simulink model "Linear_NonLinear_Model"  (R2023b)
settings: Solver=VariableStepAuto  StartTime=0.0  StopTime=400  RelTol=1e-3
undefined symbols (not defined in the file or in its folder): magnitude, P
libraries: vrlib x21
settings Model: Creator=pinki  LastModifiedBy=pinki

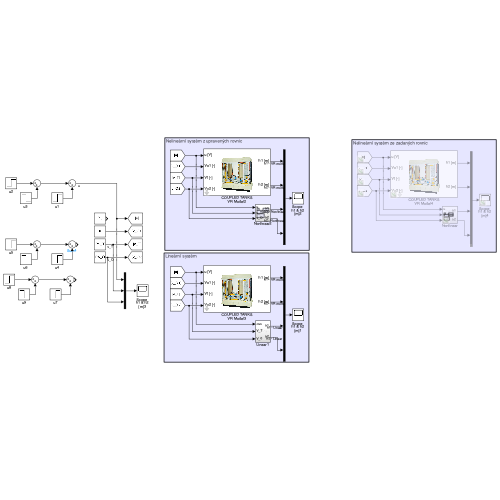
[thumbnail: Simulink's stored preview of the top-level diagram]
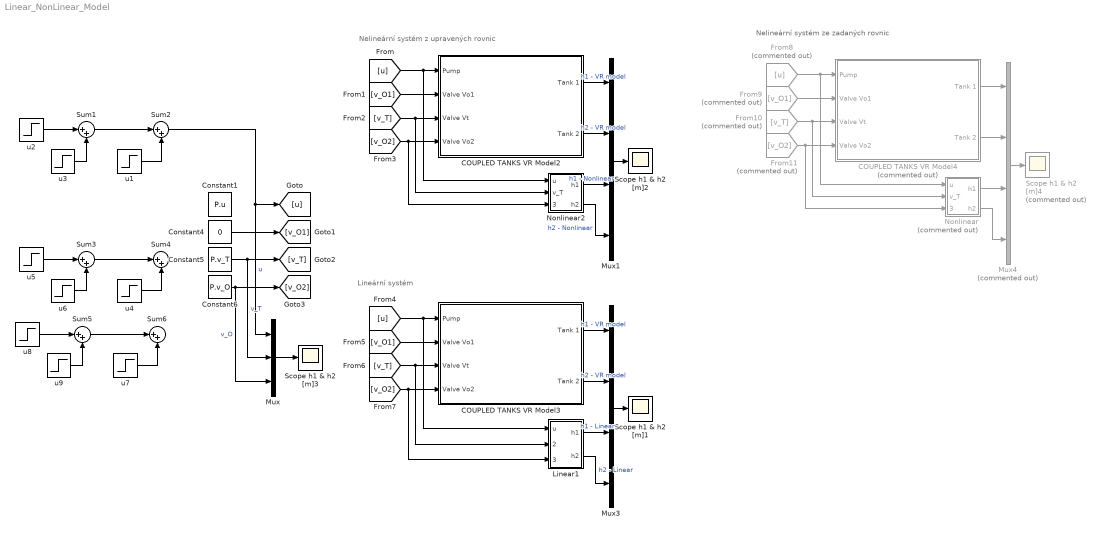
== system Linear_NonLinear_Model ==
  note: Lineární systém
  note: Nelineární systém z upravených rovnic
  note: Nelineární systém ze zadaných rovnic
  COUPLED TANKS VR Model2 : Subsystem  mask(Coupled Tanks (CT) in laboratory K26){showVR=off, sfcnParam1=P.h1, sfcnParam2=P.h2}
      mask prompts: showVR "Show VirtualWorld?"; sfcnParam1 "Initial fluid level in the left tank 1   h1(0)  [cm]"; sfcnParam2 "Initial fluid  level in the right tank 2   h2 (0) [cm]"
      mask help:
      | Coupled Tanks (CT) in laboratory K26 - Virtual Reality
      | Real-Time Workshop generated S-function.
      mask Help:
      | Couple Tanks in laboratory K26 - Virtual Reality. <br><br>
      | 
      | 
      | This is a&nbsp;virtual model of the Coupled Tanks apparatus in Laboratory of automatic control
      | theory&nbsp;26 (<a href="http://support.dce.felk.cvut.cz/lab26/" target="_blank">http://support.dce.felk.cvut.cz/lab26/</a>),
      | which consists of a&nbsp;gear-pump, two tanks (left and right), inflow and outflow pipes and transfer (V<sub>t</sub>) and
      | output valves (V<sub>o1</sub>, V<sub>o2</sub>). The&nbsp;left tank is filled with the&nbsp;fluid by the&nbsp;gear-pump
      | controller by the&nbsp;voltage&nbsp;<em>u</em>&nbsp;[V]. The&nbsp;fluid can drain from the&nbsp;left tank through
      | the&nbsp;valve&nbsp;<em>v</em><sub>o1</sub>&nbsp;[%] or can drain to the&nbsp;right tank through the&nbsp;transfer
      | valve&nbsp;<em>v</em><sub>t</sub>&nbsp;[%]. The&nbsp;fluid drains away from the&nbsp;right tank through
      | the&nbsp;valve&nbsp;<em>v</em><sub>o2</sub>&nbsp;[%].<br><br>
      | 
      | The&nbsp;system input are the&nbsp;voltage of the&nbsp;motor of the&nbsp;gear-pump&nbsp;<em>u</em>&nbsp;[V]
      | and the&nbsp;opening of
      | the&nbsp;valves&nbsp;<em>v</em><sub>o1</sub>,&nbsp;<em>v</em><sub>t</sub>,&nbsp;<em>v</em><sub>o2</sub>&nbsp;[%].
      | The&nbsp;system outputs are the&nbsp;levels of the&nbsp;fluid in
      | the&nbsp;tanks&nbsp;<em>h</em><sub>1</sub>,&nbsp;<em>h</em><sub>2</sub>&nbsp;[cm].
      | The&nbsp;dynamics of the&nbsp;gear-pump is neglected. More information can be found on the&nbsp;website
      | <a href="http://support.dce.felk.cvut.cz/lab26/" target="_blank">http://support.dce.felk.cvut.cz/lab26/</a>.<br><br>
      | 
      | 
      | In the mask of the model, it can be set:
      | <ul>
      | <li>Initial fluid level in the left tank</li>
      | <li>Initial fluid level in the right tank.</li>
      | </ul><br><br>
      | 
      | 
      | Copyright: 2008, Jan Kricka, Jirka Roubal, Petr Husek.
      mask Callback showVR:
      | if strcmp('off',get_param(gcb,'showVR'))
      |     vrclose all;
      | else
      |     if exist('figureVR')==0
      |         figureVR = vrfigure;
      |     end
      |     if exist('worldVR')==0
      |         worldVR = vrworld('CoupledTanks_VR.WRL');
      |     end
      | 	if isvalid(figureVR)==0
      |         open(worldVR);
      |         figureVR = vrfigure(worldVR,[650 80 550 350]);
      | 	end
      | end
      mask Display:
      | image(imread('CoupledTanks_Image.jpg'));
      | port_label ('input',1,'u [V]');
      | port_label ('input',2,'Vo1 [-]');
      | port_label ('input',3,'Vt [-]');
      | port_label ('input',4,'Vo2 [-]');
      | port_label ('output',1,'h1 [m]');
      | port_label ('output',2,'h2 [m]');
  COUPLED TANKS VR Model3 : Subsystem  mask(Coupled Tanks (CT) in laboratory K26){showVR=off, sfcnParam1=P.h1, sfcnParam2=P.h2}
      mask prompts: showVR "Show VirtualWorld?"; sfcnParam1 "Initial fluid level in the left tank 1   h1(0)  [cm]"; sfcnParam2 "Initial fluid  level in the right tank 2   h2 (0) [cm]"
      mask help:
      | Coupled Tanks (CT) in laboratory K26 - Virtual Reality
      | Real-Time Workshop generated S-function.
      mask Help:
      | Couple Tanks in laboratory K26 - Virtual Reality. <br><br>
      | 
      | 
      | This is a&nbsp;virtual model of the Coupled Tanks apparatus in Laboratory of automatic control
      | theory&nbsp;26 (<a href="http://support.dce.felk.cvut.cz/lab26/" target="_blank">http://support.dce.felk.cvut.cz/lab26/</a>),
      | which consists of a&nbsp;gear-pump, two tanks (left and right), inflow and outflow pipes and transfer (V<sub>t</sub>) and
      | output valves (V<sub>o1</sub>, V<sub>o2</sub>). The&nbsp;left tank is filled with the&nbsp;fluid by the&nbsp;gear-pump
      | controller by the&nbsp;voltage&nbsp;<em>u</em>&nbsp;[V]. The&nbsp;fluid can drain from the&nbsp;left tank through
      | the&nbsp;valve&nbsp;<em>v</em><sub>o1</sub>&nbsp;[%] or can drain to the&nbsp;right tank through the&nbsp;transfer
      | valve&nbsp;<em>v</em><sub>t</sub>&nbsp;[%]. The&nbsp;fluid drains away from the&nbsp;right tank through
      | the&nbsp;valve&nbsp;<em>v</em><sub>o2</sub>&nbsp;[%].<br><br>
      | 
      | The&nbsp;system input are the&nbsp;voltage of the&nbsp;motor of the&nbsp;gear-pump&nbsp;<em>u</em>&nbsp;[V]
      | and the&nbsp;opening of
      | the&nbsp;valves&nbsp;<em>v</em><sub>o1</sub>,&nbsp;<em>v</em><sub>t</sub>,&nbsp;<em>v</em><sub>o2</sub>&nbsp;[%].
      | The&nbsp;system outputs are the&nbsp;levels of the&nbsp;fluid in
      | the&nbsp;tanks&nbsp;<em>h</em><sub>1</sub>,&nbsp;<em>h</em><sub>2</sub>&nbsp;[cm].
      | The&nbsp;dynamics of the&nbsp;gear-pump is neglected. More information can be found on the&nbsp;website
      | <a href="http://support.dce.felk.cvut.cz/lab26/" target="_blank">http://support.dce.felk.cvut.cz/lab26/</a>.<br><br>
      | 
      | 
      | In the mask of the model, it can be set:
      | <ul>
      | <li>Initial fluid level in the left tank</li>
      | <li>Initial fluid level in the right tank.</li>
      | </ul><br><br>
      | 
      | 
      | Copyright: 2008, Jan Kricka, Jirka Roubal, Petr Husek.
      mask Callback showVR:
      | if strcmp('off',get_param(gcb,'showVR'))
      |     vrclose all;
      | else
      |     if exist('figureVR')==0
      |         figureVR = vrfigure;
      |     end
      |     if exist('worldVR')==0
      |         worldVR = vrworld('CoupledTanks_VR.WRL');
      |     end
      | 	if isvalid(figureVR)==0
      |         open(worldVR);
      |         figureVR = vrfigure(worldVR,[650 80 550 350]);
      | 	end
      | end
      mask Display:
      | image(imread('CoupledTanks_Image.jpg'));
      | port_label ('input',1,'u [V]');
      | port_label ('input',2,'Vo1 [-]');
      | port_label ('input',3,'Vt [-]');
      | port_label ('input',4,'Vo2 [-]');
      | port_label ('output',1,'h1 [m]');
      | port_label ('output',2,'h2 [m]');
  COUPLED TANKS VR Model4 : Subsystem  Commented=on  mask(Coupled Tanks (CT) in laboratory K26){showVR=off, sfcnParam1=P.h1, sfcnParam2=P.h2}
      mask prompts: showVR "Show VirtualWorld?"; sfcnParam1 "Initial fluid level in the left tank 1   h1(0)  [cm]"; sfcnParam2 "Initial fluid  level in the right tank 2   h2 (0) [cm]"
      mask help:
      | Coupled Tanks (CT) in laboratory K26 - Virtual Reality
      | Real-Time Workshop generated S-function.
      mask Help:
      | Couple Tanks in laboratory K26 - Virtual Reality. <br><br>
      | 
      | 
      | This is a&nbsp;virtual model of the Coupled Tanks apparatus in Laboratory of automatic control
      | theory&nbsp;26 (<a href="http://support.dce.felk.cvut.cz/lab26/" target="_blank">http://support.dce.felk.cvut.cz/lab26/</a>),
      | which consists of a&nbsp;gear-pump, two tanks (left and right), inflow and outflow pipes and transfer (V<sub>t</sub>) and
      | output valves (V<sub>o1</sub>, V<sub>o2</sub>). The&nbsp;left tank is filled with the&nbsp;fluid by the&nbsp;gear-pump
      | controller by the&nbsp;voltage&nbsp;<em>u</em>&nbsp;[V]. The&nbsp;fluid can drain from the&nbsp;left tank through
      | the&nbsp;valve&nbsp;<em>v</em><sub>o1</sub>&nbsp;[%] or can drain to the&nbsp;right tank through the&nbsp;transfer
      | valve&nbsp;<em>v</em><sub>t</sub>&nbsp;[%]. The&nbsp;fluid drains away from the&nbsp;right tank through
      | the&nbsp;valve&nbsp;<em>v</em><sub>o2</sub>&nbsp;[%].<br><br>
      | 
      | The&nbsp;system input are the&nbsp;voltage of the&nbsp;motor of the&nbsp;gear-pump&nbsp;<em>u</em>&nbsp;[V]
      | and the&nbsp;opening of
      | the&nbsp;valves&nbsp;<em>v</em><sub>o1</sub>,&nbsp;<em>v</em><sub>t</sub>,&nbsp;<em>v</em><sub>o2</sub>&nbsp;[%].
      | The&nbsp;system outputs are the&nbsp;levels of the&nbsp;fluid in
      | the&nbsp;tanks&nbsp;<em>h</em><sub>1</sub>,&nbsp;<em>h</em><sub>2</sub>&nbsp;[cm].
      | The&nbsp;dynamics of the&nbsp;gear-pump is neglected. More information can be found on the&nbsp;website
      | <a href="http://support.dce.felk.cvut.cz/lab26/" target="_blank">http://support.dce.felk.cvut.cz/lab26/</a>.<br><br>
      | 
      | 
      | In the mask of the model, it can be set:
      | <ul>
      | <li>Initial fluid level in the left tank</li>
      | <li>Initial fluid level in the right tank.</li>
      | </ul><br><br>
      | 
      | 
      | Copyright: 2008, Jan Kricka, Jirka Roubal, Petr Husek.
      mask Callback showVR:
      | if strcmp('off',get_param(gcb,'showVR'))
      |     vrclose all;
      | else
      |     if exist('figureVR')==0
      |         figureVR = vrfigure;
      |     end
      |     if exist('worldVR')==0
      |         worldVR = vrworld('CoupledTanks_VR.WRL');
      |     end
      | 	if isvalid(figureVR)==0
      |         open(worldVR);
      |         figureVR = vrfigure(worldVR,[650 80 550 350]);
      | 	end
      | end
      mask Display:
      | image(imread('CoupledTanks_Image.jpg'));
      | port_label ('input',1,'u [V]');
      | port_label ('input',2,'Vo1 [-]');
      | port_label ('input',3,'Vt [-]');
      | port_label ('input',4,'Vo2 [-]');
      | port_label ('output',1,'h1 [m]');
      | port_label ('output',2,'h2 [m]');
  Constant1 : Constant  Value=P.u
  Constant4 : Constant  Value=0
  Constant5 : Constant  Value=P.v_T
  Constant6 : Constant  Value=P.v_O
  From10 : From  Commented=on  GotoTag=v_T
  From11 : From  Commented=on  GotoTag=v_O2
  From8 : From  Commented=on  GotoTag=u
  From9 : From  Commented=on  GotoTag=v_O1
  Linear1 : Subsystem
  Mux : Mux  Inputs=3
  Mux1 : Mux
  Mux3 : Mux
  Mux4 : Mux  Commented=on
  Nonlinear : Subsystem  Commented=on
  Nonlinear2 : Subsystem
  Scope h1 & h2 [m]1 : Scope
  Scope h1 & h2 [m]2 : Scope
  Scope h1 & h2 [m]3 : Scope
  Scope h1 & h2 [m]4 : Scope  Commented=on
  Sum{1..6} (6 alike) : Sum  Inputs=|++
  u1 : Step  Time=300  After=2  SampleTime=0
  u2 : Step  Time=100  Before=P.u  After=P.u+0.5  SampleTime=0
  u3 : Step  Time=200  After=-1  SampleTime=0
  u4 : Step  Time=300  After=0.4  SampleTime=0
  u5 : Step  Time=100  Before=P.v_T  After=P.v_T+0.1  SampleTime=0
  u6 : Step  Time=200  After=-0.2  SampleTime=0
  u7 : Step  Time=300  After=0.4  SampleTime=0
  u8 : Step  Time=100  Before=P.v_O  After=P.v_O+0.1  SampleTime=0
  u9 : Step  Time=200  After=-0.2  SampleTime=0
  wires:
  [v_O2] -> Nonlinear2/3(v_O), COUPLED TANKS VR Model2/4(Valve Vo2)
  COUPLED TANKS VR Model2/1(Tank 1) -> Mux1/1  "h1 - VR model"
  Sum1/1 -> Sum2/1
  u1/1 -> Sum2/2
  [v_O1] -> COUPLED TANKS VR Model2/2(Valve Vo1)
  u3/1 -> Sum1/2
  [v_T] -> COUPLED TANKS VR Model2/3(Valve Vt), Nonlinear2/2(v_T)
  Mux1/1 -> Scope h1 & h2 [m]2/1
  COUPLED TANKS VR Model2/2(Tank 2) -> Mux1/2  "h2 - VR model"
  u2/1 -> Sum1/1
  Nonlinear2/1(h1) -> Mux1/3  "h1 - Nonlinear"
  Nonlinear2/2(h2) -> Mux1/4  "h2 - Nonlinear"
  [u] -> Nonlinear2/1(u), COUPLED TANKS VR Model2/1(Pump)
  Constant4/1 -> [v_O1]
  [v_T] -> Linear1/2(V_T), COUPLED TANKS VR Model3/3(Valve Vt)
  COUPLED TANKS VR Model3/1(Tank 1) -> Mux3/1  "h1 - VR model"
  Linear1/2(h2) -> Mux3/4  "h2 - Linear"
  Linear1/1(h1) -> Mux3/3  "h1 - Linear"
  Mux3/1 -> Scope h1 & h2 [m]1/1
  COUPLED TANKS VR Model3/2(Tank 2) -> Mux3/2  "h2 - VR model"
  [u] -> Linear1/1(u), COUPLED TANKS VR Model3/1(Pump)
  [v_O2] -> Linear1/3(V_0), COUPLED TANKS VR Model3/4(Valve Vo2)
  [v_O1] -> COUPLED TANKS VR Model3/2(Valve Vo1)
  Mux4/1 -> Scope h1 & h2 [m]4/1
  COUPLED TANKS VR Model4/2(Tank 2) -> Mux4/2
  Nonlinear/1(h1) -> Mux4/3
  Nonlinear/2(h2) -> Mux4/4
  From8/1 -> Nonlinear/1(u), COUPLED TANKS VR Model4/1(Pump)
  COUPLED TANKS VR Model4/1(Tank 1) -> Mux4/1
  From11/1 -> Nonlinear/3(v_O), COUPLED TANKS VR Model4/4(Valve Vo2)
  From10/1 -> Nonlinear/2(v_T), COUPLED TANKS VR Model4/3(Valve Vt)
  From9/1 -> COUPLED TANKS VR Model4/2(Valve Vo1)
  Sum3/1 -> Sum4/1
  u4/1 -> Sum4/2
  u6/1 -> Sum3/2
  u5/1 -> Sum3/1
  Mux/1 -> Scope h1 & h2 [m]3/1
  Sum5/1 -> Sum6/1
  u7/1 -> Sum6/2
  u8/1 -> Sum5/1
  u9/1 -> Sum5/2
  Constant6/1 -> Mux/3, [v_O2]  "v_O"
  Constant5/1 -> Mux/2, [v_T]  "v_T"
  Sum2/1 -> [u], Mux/1  "u"

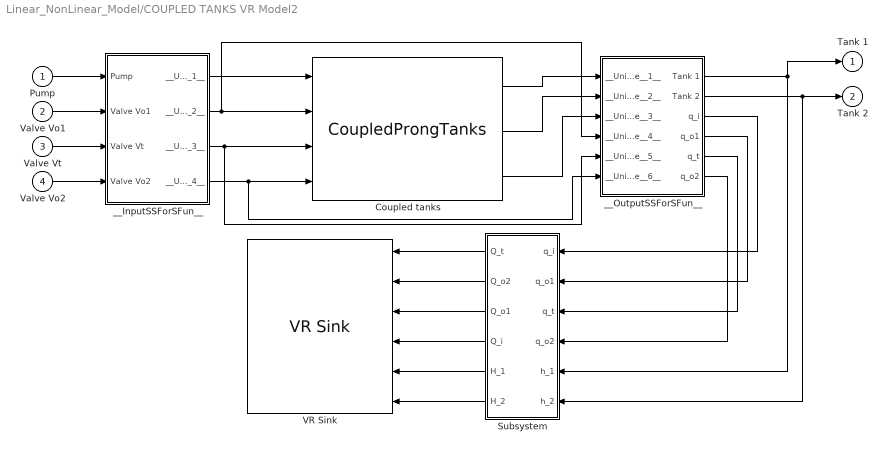
== system Linear_NonLinear_Model/COUPLED TANKS VR Model2 ==
  Pump : Inport
  Valve Vo1 : Inport  Port=2
  Valve Vt : Inport  Port=3
  Valve Vo2 : Inport  Port=4
  Coupled tanks : M-S-Function  FunctionName=CoupledProngTanks  Parameters=h10 h20  mask{h10=sfcnParam1, h20=sfcnParam2}
      mask prompts: h10 "h1_init"; h20 "h2_init"
      mask Display:
      | port_label('input',1,'Pump');
      | port_label('input',2,'Valve Vo1');
      | port_label('input',3,'Valve Vt');
      | port_label('input',4,'Valve Vo2');
      | port_label('output',1,'Tank 1');
      | port_label('output',2,'Tank 2');
      | port_label('output',3,'q_i');
  Subsystem : Subsystem
  VR Sink : vrlib/VR Sink  InstantiateOnLoad=on  SampleTime=-1  ViewEnable=on  RemoteChange=off  RemoteView=on  FieldsWritten=Valve_t.rotation.4.1.double#Valve_o2.rotation.4.1.double#Valve_o1.rotation.4.1.double#Pump.rotation.4.1.double#water1.scale.3.1.double#water2.scale.3.1.double  WorldFileName=CoupledTanks_VR.WRL  AutoView=off  VideoDimensions=[]  AllowVariableSize=off
  __InputSSForSFun__ : Subsystem
  __OutputSSForSFun__ : Subsystem
  Tank 1 : Outport  OutDataTypeStr=double  PortDimensions=1  SampleTime=[-1 0]
  Tank 2 : Outport  Port=2  OutDataTypeStr=double  PortDimensions=1  SampleTime=[-1 0]
  wires:
  __OutputSSForSFun__/6(q_o2) -> Subsystem/4(q_o2)
  __OutputSSForSFun__/5(q_t) -> Subsystem/3(q_t)
  __OutputSSForSFun__/4(q_o1) -> Subsystem/2(q_o1)
  __OutputSSForSFun__/3(q_i) -> Subsystem/1(q_i)
  Subsystem/2(Q_o2) -> VR Sink/2
  Subsystem/3(Q_o1) -> VR Sink/3
  Subsystem/4(Q_i) -> VR Sink/4
  Subsystem/1(Q_t) -> VR Sink/1
  Subsystem/6(H_2) -> VR Sink/6
  Subsystem/5(H_1) -> VR Sink/5
  __OutputSSForSFun__/2(Tank 2) -> Subsystem/6(h_2), Tank 2/1
  __OutputSSForSFun__/1(Tank 1) -> Tank 1/1, Subsystem/5(h_1)
  __InputSSForSFun__/4(__UniqueOutportName__4__) -> __OutputSSForSFun__/6(__UniqueInportName__6__), Coupled tanks/4
  __InputSSForSFun__/3(__UniqueOutportName__3__) -> __OutputSSForSFun__/5(__UniqueInportName__5__), Coupled tanks/3
  Coupled tanks/2 -> __OutputSSForSFun__/2(__UniqueInportName__2__)
  Coupled tanks/1 -> __OutputSSForSFun__/1(__UniqueInportName__1__)
  __InputSSForSFun__/2(__UniqueOutportName__2__) -> __OutputSSForSFun__/4(__UniqueInportName__4__), Coupled tanks/2
  __InputSSForSFun__/1(__UniqueOutportName__1__) -> Coupled tanks/1
  Valve Vo2/1 -> __InputSSForSFun__/4(Valve Vo2)
  Valve Vt/1 -> __InputSSForSFun__/3(Valve Vt)
  Valve Vo1/1 -> __InputSSForSFun__/2(Valve Vo1)
  Pump/1 -> __InputSSForSFun__/1(Pump)
  Coupled tanks/3 -> __OutputSSForSFun__/3(__UniqueInportName__3__)

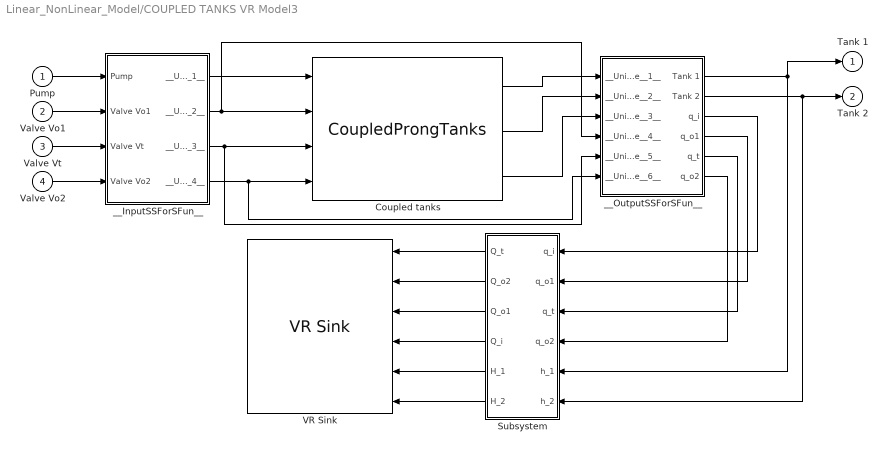
== system Linear_NonLinear_Model/COUPLED TANKS VR Model3 ==
  Pump : Inport
  Valve Vo1 : Inport  Port=2
  Valve Vt : Inport  Port=3
  Valve Vo2 : Inport  Port=4
  Coupled tanks : M-S-Function  FunctionName=CoupledProngTanks  Parameters=h10 h20  mask{h10=sfcnParam1, h20=sfcnParam2}
      mask prompts: h10 "h1_init"; h20 "h2_init"
      mask Display:
      | port_label('input',1,'Pump');
      | port_label('input',2,'Valve Vo1');
      | port_label('input',3,'Valve Vt');
      | port_label('input',4,'Valve Vo2');
      | port_label('output',1,'Tank 1');
      | port_label('output',2,'Tank 2');
      | port_label('output',3,'q_i');
  Subsystem : Subsystem
  VR Sink : vrlib/VR Sink  InstantiateOnLoad=on  SampleTime=-1  ViewEnable=on  RemoteChange=off  RemoteView=on  FieldsWritten=Valve_t.rotation.4.1.double#Valve_o2.rotation.4.1.double#Valve_o1.rotation.4.1.double#Pump.rotation.4.1.double#water1.scale.3.1.double#water2.scale.3.1.double  WorldFileName=CoupledTanks_VR.WRL  AutoView=off  VideoDimensions=[]  AllowVariableSize=off
  __InputSSForSFun__ : Subsystem
  __OutputSSForSFun__ : Subsystem
  Tank 1 : Outport  OutDataTypeStr=double  PortDimensions=1  SampleTime=[-1 0]
  Tank 2 : Outport  Port=2  OutDataTypeStr=double  PortDimensions=1  SampleTime=[-1 0]
  wires:
  __OutputSSForSFun__/6(q_o2) -> Subsystem/4(q_o2)
  __OutputSSForSFun__/5(q_t) -> Subsystem/3(q_t)
  __OutputSSForSFun__/4(q_o1) -> Subsystem/2(q_o1)
  __OutputSSForSFun__/3(q_i) -> Subsystem/1(q_i)
  Subsystem/2(Q_o2) -> VR Sink/2
  Subsystem/3(Q_o1) -> VR Sink/3
  Subsystem/4(Q_i) -> VR Sink/4
  Subsystem/1(Q_t) -> VR Sink/1
  Subsystem/6(H_2) -> VR Sink/6
  Subsystem/5(H_1) -> VR Sink/5
  __OutputSSForSFun__/2(Tank 2) -> Subsystem/6(h_2), Tank 2/1
  __OutputSSForSFun__/1(Tank 1) -> Tank 1/1, Subsystem/5(h_1)
  __InputSSForSFun__/4(__UniqueOutportName__4__) -> __OutputSSForSFun__/6(__UniqueInportName__6__), Coupled tanks/4
  __InputSSForSFun__/3(__UniqueOutportName__3__) -> __OutputSSForSFun__/5(__UniqueInportName__5__), Coupled tanks/3
  Coupled tanks/2 -> __OutputSSForSFun__/2(__UniqueInportName__2__)
  Coupled tanks/1 -> __OutputSSForSFun__/1(__UniqueInportName__1__)
  __InputSSForSFun__/2(__UniqueOutportName__2__) -> __OutputSSForSFun__/4(__UniqueInportName__4__), Coupled tanks/2
  __InputSSForSFun__/1(__UniqueOutportName__1__) -> Coupled tanks/1
  Valve Vo2/1 -> __InputSSForSFun__/4(Valve Vo2)
  Valve Vt/1 -> __InputSSForSFun__/3(Valve Vt)
  Valve Vo1/1 -> __InputSSForSFun__/2(Valve Vo1)
  Pump/1 -> __InputSSForSFun__/1(Pump)
  Coupled tanks/3 -> __OutputSSForSFun__/3(__UniqueInportName__3__)

== system Linear_NonLinear_Model/COUPLED TANKS VR Model4 ==
  Pump : Inport
  Valve Vo1 : Inport  Port=2
  Valve Vt : Inport  Port=3
  Valve Vo2 : Inport  Port=4
  Coupled tanks : M-S-Function  FunctionName=CoupledProngTanks  Parameters=h10 h20  mask{h10=sfcnParam1, h20=sfcnParam2}
      mask prompts: h10 "h1_init"; h20 "h2_init"
      mask Display:
      | port_label('input',1,'Pump');
      | port_label('input',2,'Valve Vo1');
      | port_label('input',3,'Valve Vt');
      | port_label('input',4,'Valve Vo2');
      | port_label('output',1,'Tank 1');
      | port_label('output',2,'Tank 2');
      | port_label('output',3,'q_i');
  Subsystem : Subsystem
  VR Sink : vrlib/VR Sink  InstantiateOnLoad=on  SampleTime=-1  ViewEnable=on  RemoteChange=off  RemoteView=on  FieldsWritten=Valve_t.rotation.4.1.double#Valve_o2.rotation.4.1.double#Valve_o1.rotation.4.1.double#Pump.rotation.4.1.double#water1.scale.3.1.double#water2.scale.3.1.double  WorldFileName=CoupledTanks_VR.WRL  AutoView=off  VideoDimensions=[]  AllowVariableSize=off
  __InputSSForSFun__ : Subsystem
  __OutputSSForSFun__ : Subsystem
  Tank 1 : Outport  OutDataTypeStr=double  PortDimensions=1  SampleTime=[-1 0]
  Tank 2 : Outport  Port=2  OutDataTypeStr=double  PortDimensions=1  SampleTime=[-1 0]
  wires:
  __OutputSSForSFun__/6(q_o2) -> Subsystem/4(q_o2)
  __OutputSSForSFun__/5(q_t) -> Subsystem/3(q_t)
  __OutputSSForSFun__/4(q_o1) -> Subsystem/2(q_o1)
  __OutputSSForSFun__/3(q_i) -> Subsystem/1(q_i)
  Subsystem/2(Q_o2) -> VR Sink/2
  Subsystem/3(Q_o1) -> VR Sink/3
  Subsystem/4(Q_i) -> VR Sink/4
  Subsystem/1(Q_t) -> VR Sink/1
  Subsystem/6(H_2) -> VR Sink/6
  Subsystem/5(H_1) -> VR Sink/5
  __OutputSSForSFun__/2(Tank 2) -> Subsystem/6(h_2), Tank 2/1
  __OutputSSForSFun__/1(Tank 1) -> Tank 1/1, Subsystem/5(h_1)
  __InputSSForSFun__/4(__UniqueOutportName__4__) -> __OutputSSForSFun__/6(__UniqueInportName__6__), Coupled tanks/4
  __InputSSForSFun__/3(__UniqueOutportName__3__) -> __OutputSSForSFun__/5(__UniqueInportName__5__), Coupled tanks/3
  Coupled tanks/2 -> __OutputSSForSFun__/2(__UniqueInportName__2__)
  Coupled tanks/1 -> __OutputSSForSFun__/1(__UniqueInportName__1__)
  __InputSSForSFun__/2(__UniqueOutportName__2__) -> __OutputSSForSFun__/4(__UniqueInportName__4__), Coupled tanks/2
  __InputSSForSFun__/1(__UniqueOutportName__1__) -> Coupled tanks/1
  Valve Vo2/1 -> __InputSSForSFun__/4(Valve Vo2)
  Valve Vt/1 -> __InputSSForSFun__/3(Valve Vt)
  Valve Vo1/1 -> __InputSSForSFun__/2(Valve Vo1)
  Pump/1 -> __InputSSForSFun__/1(Pump)
  Coupled tanks/3 -> __OutputSSForSFun__/3(__UniqueInportName__3__)

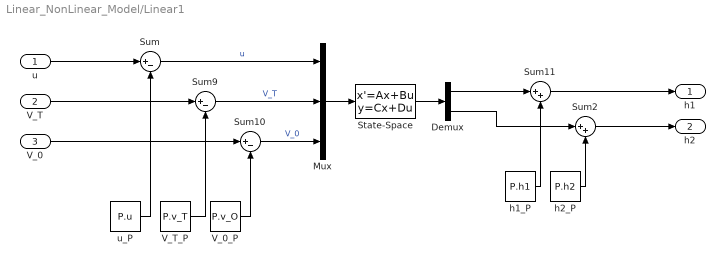
== system Linear_NonLinear_Model/Linear1 ==
  u : Inport
  V_T : Inport  Port=2
  V_0 : Inport  Port=3
  Demux : Demux  Outputs=2
  Mux : Mux  Inputs=3
  State-Space : StateSpace  A=P.A  B=P.B  C=P.C  D=P.D  InitialCondition=0
  Sum : Sum  Inputs=|+-
  Sum10 : Sum  Inputs=|+-
  Sum11 : Sum  Inputs=|++
  Sum2 : Sum  Inputs=|++
  Sum9 : Sum  Inputs=|+-
  V_0_P : Constant  Value=P.v_O
  V_T_P : Constant  Value=P.v_T
  h1_P : Constant  Value=P.h1
  h2_P : Constant  Value=P.h2
  u_P : Constant  Value=P.u
  h1 : Outport
  h2 : Outport  Port=2
  wires:
  u/1 -> Sum/1
  V_0/1 -> Sum10/1
  State-Space/1 -> Demux/1
  V_T/1 -> Sum9/1
  Sum9/1 -> Mux/2  "V_T"
  Sum/1 -> Mux/1  "u"
  Demux/2 -> Sum2/1
  h1_P/1 -> Sum11/2
  h2_P/1 -> Sum2/2
  Sum11/1 -> h1/1
  V_0_P/1 -> Sum10/2
  V_T_P/1 -> Sum9/2
  Sum10/1 -> Mux/3  "V_0"
  Mux/1 -> State-Space/1
  Demux/1 -> Sum11/1
  u_P/1 -> Sum/2
  Sum2/1 -> h2/1

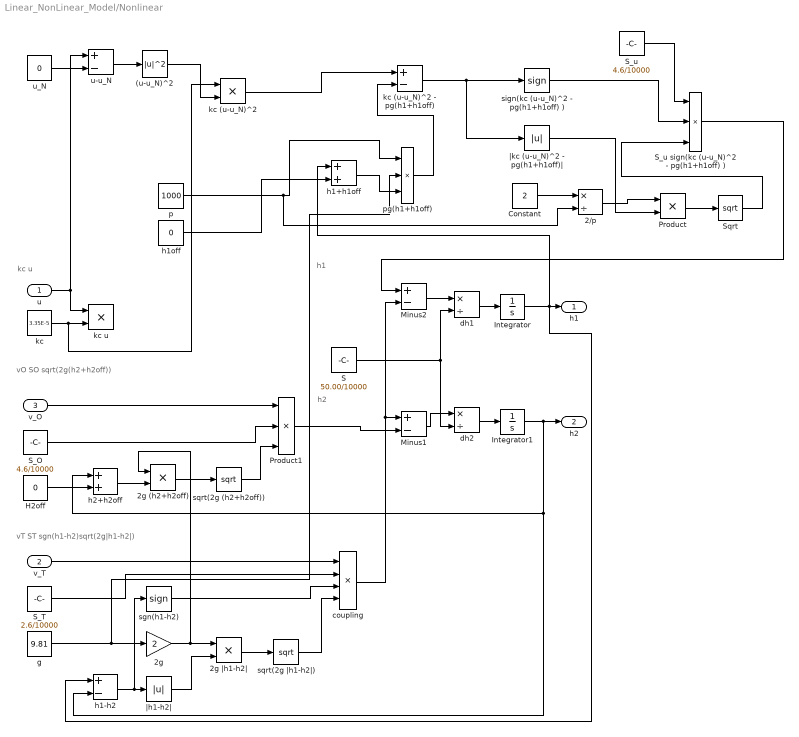
== system Linear_NonLinear_Model/Nonlinear ==
  note: h1
  note: h2
  note: vO SO sqrt(2g(h2+h2off))
  note: vT ST sgn(h1-h2)sqrt(2g|h1-h2|)
  note: kc u
  u : Inport
  v_T : Inport  Port=2
  v_O : Inport  Port=3
  (u-u_N)^2 : Math  Operator=magnitude^2
  2/p : Product  Inputs=*/
  2g : Gain  Gain=2
  2g (h2+h2off) : Product
  2g |h1-h2| : Product
  Constant : Constant  Value=2
  H2off : Constant  Value=0
  Integrator : Integrator  InitialCondition=P.h1
  Integrator1 : Integrator  InitialCondition=P.h2
  Minus1 : Sum  Inputs=+-
  Minus2 : Sum  Inputs=+-
  Product : Product
  Product1 : Product  Inputs=3
  S : Constant  Value=50.00/10000
  S_O : Constant  Value=4.6/10000
  S_T : Constant  Value=2.6/10000
  S_u : Constant  Value=4.6/10000
  S_u sign(kc (u-u_N)^2 - pg(h1+h1off) ) : Product  Inputs=3
  Sqrt : Sqrt
  coupling : Product  Inputs=4
  dh1 : Product  Inputs=*/
  dh2 : Product  Inputs=*/
  g : Constant  Value=9.81
  h1+h1off : Sum
  h1-h2 : Sum  Inputs=+-
  h1off : Constant  Value=0
  h2+h2off : Sum
  kc : Constant  Value=3.35E-5
  kc (u-u_N)^2 : Product
  "kc (u-u_N)^2 - pg(h1+h1off) " : Sum  Inputs=+-
  kc u : Product
  p : Constant  Value=1000
  pg(h1+h1off) : Product  Inputs=3
  sgn(h1-h2) : Signum
  sign(kc (u-u_N)^2 - pg(h1+h1off) ) : Signum
  sqrt(2g (h2+h2off)) : Sqrt
  sqrt(2g |h1-h2|) : Sqrt
  u-u_N : Sum  Inputs=+-
  u_N : Constant  Value=0
  |h1-h2| : Abs  SaturateOnIntegerOverflow=off
  |kc (u-u_N)^2 - pg(h1+h1off)| : Abs  SaturateOnIntegerOverflow=off
  h1 : Outport
  h2 : Outport  Port=2
  wires:
  v_O/1 -> Product1/1
  sgn(h1-h2)/1 -> coupling/3
  |h1-h2|/1 -> 2g |h1-h2|/2
  h2+h2off/1 -> 2g (h2+h2off)/2
  Product1/1 -> Minus1/2
  S_O/1 -> Product1/2
  Integrator1/1 -> h2/1, h2+h2off/1, h1-h2/2
  S/1 -> dh1/2, dh2/2
  S_T/1 -> coupling/2
  dh1/1 -> Integrator/1
  h1-h2/1 -> |h1-h2|/1, sgn(h1-h2)/1
  Minus2/1 -> dh1/1
  u/1 -> kc u/1, u-u_N/1
  v_T/1 -> coupling/1
  H2off/1 -> h2+h2off/2
  sqrt(2g |h1-h2|)/1 -> coupling/4
  2g/1 -> 2g |h1-h2|/1, 2g (h2+h2off)/1
  kc/1 -> kc (u-u_N)^2/1, kc u/2
  coupling/1 -> Minus2/2, Minus1/1
  Integrator/1 -> h1+h1off/1, h1/1, h1-h2/1
  Minus1/1 -> dh2/1
  2g |h1-h2|/1 -> sqrt(2g |h1-h2|)/1
  dh2/1 -> Integrator1/1
  2g (h2+h2off)/1 -> sqrt(2g (h2+h2off))/1
  sqrt(2g (h2+h2off))/1 -> Product1/3
  u_N/1 -> u-u_N/2
  u-u_N/1 -> (u-u_N)^2/1
  (u-u_N)^2/1 -> kc (u-u_N)^2/2
  h1off/1 -> h1+h1off/2
  h1+h1off/1 -> pg(h1+h1off)/3
  p/1 -> 2/p/2, pg(h1+h1off)/1
  g/1 -> pg(h1+h1off)/2, 2g/1
  kc (u-u_N)^2/1 -> "kc (u-u_N)^2 - pg(h1+h1off) "/1
  pg(h1+h1off)/1 -> "kc (u-u_N)^2 - pg(h1+h1off) "/2
  "kc (u-u_N)^2 - pg(h1+h1off) "/1 -> |kc (u-u_N)^2 - pg(h1+h1off)|/1, sign(kc (u-u_N)^2 - pg(h1+h1off) )/1
  S_u/1 -> S_u sign(kc (u-u_N)^2 - pg(h1+h1off) )/1
  sign(kc (u-u_N)^2 - pg(h1+h1off) )/1 -> S_u sign(kc (u-u_N)^2 - pg(h1+h1off) )/2
  Constant/1 -> 2/p/1
  2/p/1 -> Product/1
  |kc (u-u_N)^2 - pg(h1+h1off)|/1 -> Product/2
  Product/1 -> Sqrt/1
  Sqrt/1 -> S_u sign(kc (u-u_N)^2 - pg(h1+h1off) )/3
  S_u sign(kc (u-u_N)^2 - pg(h1+h1off) )/1 -> Minus2/1

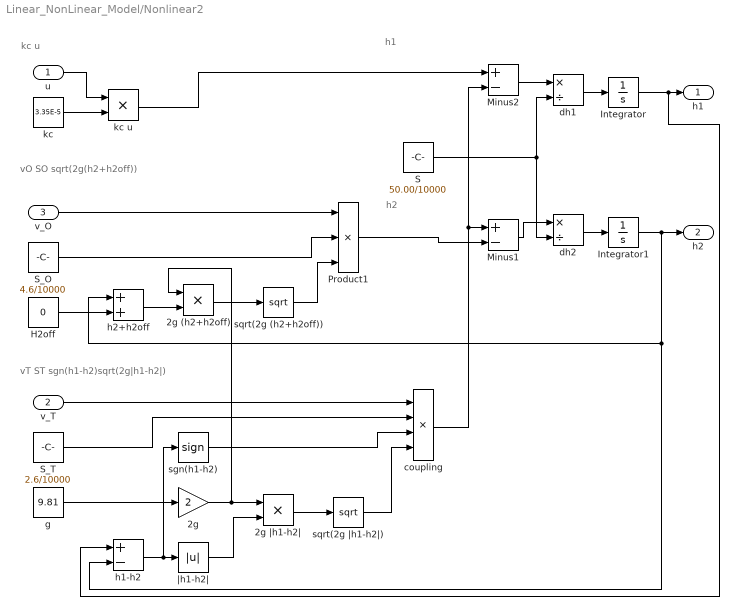
== system Linear_NonLinear_Model/Nonlinear2 ==
  note: h1
  note: h2
  note: vO SO sqrt(2g(h2+h2off))
  note: vT ST sgn(h1-h2)sqrt(2g|h1-h2|)
  note: kc u
  u : Inport
  v_T : Inport  Port=2
  v_O : Inport  Port=3
  2g : Gain  Gain=2
  2g (h2+h2off) : Product
  2g |h1-h2| : Product
  H2off : Constant  Value=0
  Integrator : Integrator  InitialCondition=P.h1
  Integrator1 : Integrator  InitialCondition=P.h2
  Minus1 : Sum  Inputs=+-
  Minus2 : Sum  Inputs=+-
  Product1 : Product  Inputs=3
  S : Constant  Value=50.00/10000
  S_O : Constant  Value=4.6/10000
  S_T : Constant  Value=2.6/10000
  coupling : Product  Inputs=4
  dh1 : Product  Inputs=*/
  dh2 : Product  Inputs=*/
  g : Constant  Value=9.81
  h1-h2 : Sum  Inputs=+-
  h2+h2off : Sum
  kc : Constant  Value=3.35E-5
  kc u : Product
  sgn(h1-h2) : Signum
  sqrt(2g (h2+h2off)) : Sqrt
  sqrt(2g |h1-h2|) : Sqrt
  |h1-h2| : Abs  SaturateOnIntegerOverflow=off
  h1 : Outport
  h2 : Outport  Port=2
  wires:
  v_O/1 -> Product1/1
  g/1 -> 2g/1
  sgn(h1-h2)/1 -> coupling/3
  |h1-h2|/1 -> 2g |h1-h2|/2
  h2+h2off/1 -> 2g (h2+h2off)/2
  Product1/1 -> Minus1/2
  S_O/1 -> Product1/2
  Integrator1/1 -> h2/1, h2+h2off/1, h1-h2/2
  S/1 -> dh1/2, dh2/2
  S_T/1 -> coupling/2
  dh1/1 -> Integrator/1
  h1-h2/1 -> |h1-h2|/1, sgn(h1-h2)/1
  Minus2/1 -> dh1/1
  kc u/1 -> Minus2/1
  u/1 -> kc u/1
  v_T/1 -> coupling/1
  H2off/1 -> h2+h2off/2
  sqrt(2g |h1-h2|)/1 -> coupling/4
  2g/1 -> 2g |h1-h2|/1, 2g (h2+h2off)/1
  kc/1 -> kc u/2
  coupling/1 -> Minus2/2, Minus1/1
  Integrator/1 -> h1/1, h1-h2/1
  Minus1/1 -> dh2/1
  2g |h1-h2|/1 -> sqrt(2g |h1-h2|)/1
  dh2/1 -> Integrator1/1
  2g (h2+h2off)/1 -> sqrt(2g (h2+h2off))/1
  sqrt(2g (h2+h2off))/1 -> Product1/3

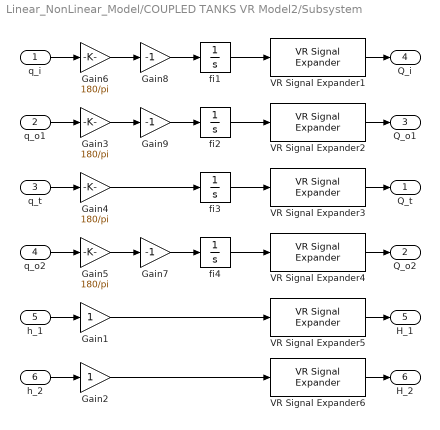
== system Linear_NonLinear_Model/COUPLED TANKS VR Model2/Subsystem ==
  q_i : Inport
  q_o1 : Inport  Port=2
  q_t : Inport  Port=3
  q_o2 : Inport  Port=4
  h_1 : Inport  Port=5
  h_2 : Inport  Port=6
  Gain1 : Gain
  Gain2 : Gain
  Gain{3..6} (4 alike) : Gain  Gain=180/pi
  Gain7 : Gain  Gain=-1
  Gain8 : Gain  Gain=-1
  Gain9 : Gain  Gain=-1
  VR Signal Expander{1..4} (4 alike) : vrlib/VR Signal Expander  outwidth=4  outidx=[4]
  VR Signal Expander5 : vrlib/VR Signal Expander  outwidth=3  outidx=[2]
  VR Signal Expander6 : vrlib/VR Signal Expander  outwidth=3  outidx=[2]
  fi{1..4} (4 alike) : Integrator
  Q_t : Outport
  Q_o2 : Outport  Port=2
  Q_o1 : Outport  Port=3
  Q_i : Outport  Port=4
  H_1 : Outport  Port=5
  H_2 : Outport  Port=6
  wires:
  Gain9/1 -> fi2/1
  Gain8/1 -> fi1/1
  Gain7/1 -> fi4/1
  Gain5/1 -> Gain7/1
  q_o2/1 -> Gain5/1
  VR Signal Expander4/1 -> Q_o2/1
  fi4/1 -> VR Signal Expander4/1
  Gain4/1 -> fi3/1
  Gain6/1 -> Gain8/1
  Gain3/1 -> Gain9/1
  q_t/1 -> Gain4/1
  q_o1/1 -> Gain3/1
  Gain2/1 -> VR Signal Expander6/1
  Gain1/1 -> VR Signal Expander5/1
  VR Signal Expander6/1 -> H_2/1
  VR Signal Expander5/1 -> H_1/1
  VR Signal Expander1/1 -> Q_i/1
  VR Signal Expander2/1 -> Q_o1/1
  VR Signal Expander3/1 -> Q_t/1
  h_2/1 -> Gain2/1
  h_1/1 -> Gain1/1
  q_i/1 -> Gain6/1
  fi2/1 -> VR Signal Expander2/1
  fi3/1 -> VR Signal Expander3/1
  fi1/1 -> VR Signal Expander1/1

== system Linear_NonLinear_Model/COUPLED TANKS VR Model2/__InputSSForSFun__ ==
  Pump : Inport
  Valve Vo1 : Inport  Port=2
  Valve Vt : Inport  Port=3
  Valve Vo2 : Inport  Port=4
  __UniqueOutportName__1__ : Outport
  __UniqueOutportName__2__ : Outport  Port=2
  __UniqueOutportName__3__ : Outport  Port=3
  __UniqueOutportName__4__ : Outport  Port=4
  wires:
  Valve Vo2/1 -> __UniqueOutportName__4__/1
  Valve Vt/1 -> __UniqueOutportName__3__/1
  Valve Vo1/1 -> __UniqueOutportName__2__/1
  Pump/1 -> __UniqueOutportName__1__/1

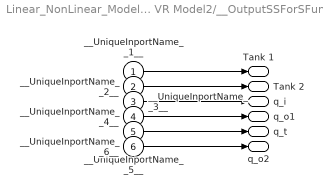
== system Linear_NonLinear_Model/COUPLED TANKS VR Model2/__OutputSSForSFun__ ==
  __UniqueInportName__1__ : Inport
  __UniqueInportName__2__ : Inport  Port=2
  __UniqueInportName__3__ : Inport  Port=3
  __UniqueInportName__4__ : Inport  Port=4
  __UniqueInportName__5__ : Inport  Port=5
  __UniqueInportName__6__ : Inport  Port=6
  Tank 1 : Outport  OutDataTypeStr=double  PortDimensions=1  SampleTime=[-1 0]
  Tank 2 : Outport  Port=2  OutDataTypeStr=double  PortDimensions=1  SampleTime=[-1 0]
  q_i : Outport  Port=3  OutDataTypeStr=double  PortDimensions=1  SampleTime=[0 1]
  q_o1 : Outport  Port=4  OutDataTypeStr=double  PortDimensions=1  SampleTime=[-1 0]
  q_t : Outport  Port=5  OutDataTypeStr=double  PortDimensions=1  SampleTime=[-1 0]
  q_o2 : Outport  Port=6  OutDataTypeStr=double  PortDimensions=1  SampleTime=[-1 0]
  wires:
  __UniqueInportName__6__/1 -> q_o2/1
  __UniqueInportName__5__/1 -> q_t/1
  __UniqueInportName__4__/1 -> q_o1/1
  __UniqueInportName__3__/1 -> q_i/1
  __UniqueInportName__2__/1 -> Tank 2/1
  __UniqueInportName__1__/1 -> Tank 1/1

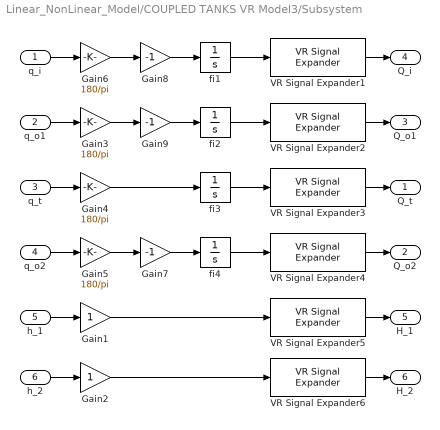
== system Linear_NonLinear_Model/COUPLED TANKS VR Model3/Subsystem ==
  q_i : Inport
  q_o1 : Inport  Port=2
  q_t : Inport  Port=3
  q_o2 : Inport  Port=4
  h_1 : Inport  Port=5
  h_2 : Inport  Port=6
  Gain1 : Gain
  Gain2 : Gain
  Gain{3..6} (4 alike) : Gain  Gain=180/pi
  Gain7 : Gain  Gain=-1
  Gain8 : Gain  Gain=-1
  Gain9 : Gain  Gain=-1
  VR Signal Expander{1..4} (4 alike) : vrlib/VR Signal Expander  outwidth=4  outidx=[4]
  VR Signal Expander5 : vrlib/VR Signal Expander  outwidth=3  outidx=[2]
  VR Signal Expander6 : vrlib/VR Signal Expander  outwidth=3  outidx=[2]
  fi{1..4} (4 alike) : Integrator
  Q_t : Outport
  Q_o2 : Outport  Port=2
  Q_o1 : Outport  Port=3
  Q_i : Outport  Port=4
  H_1 : Outport  Port=5
  H_2 : Outport  Port=6
  wires:
  Gain9/1 -> fi2/1
  Gain8/1 -> fi1/1
  Gain7/1 -> fi4/1
  Gain5/1 -> Gain7/1
  q_o2/1 -> Gain5/1
  VR Signal Expander4/1 -> Q_o2/1
  fi4/1 -> VR Signal Expander4/1
  Gain4/1 -> fi3/1
  Gain6/1 -> Gain8/1
  Gain3/1 -> Gain9/1
  q_t/1 -> Gain4/1
  q_o1/1 -> Gain3/1
  Gain2/1 -> VR Signal Expander6/1
  Gain1/1 -> VR Signal Expander5/1
  VR Signal Expander6/1 -> H_2/1
  VR Signal Expander5/1 -> H_1/1
  VR Signal Expander1/1 -> Q_i/1
  VR Signal Expander2/1 -> Q_o1/1
  VR Signal Expander3/1 -> Q_t/1
  h_2/1 -> Gain2/1
  h_1/1 -> Gain1/1
  q_i/1 -> Gain6/1
  fi2/1 -> VR Signal Expander2/1
  fi3/1 -> VR Signal Expander3/1
  fi1/1 -> VR Signal Expander1/1

== system Linear_NonLinear_Model/COUPLED TANKS VR Model3/__InputSSForSFun__ ==
  Pump : Inport
  Valve Vo1 : Inport  Port=2
  Valve Vt : Inport  Port=3
  Valve Vo2 : Inport  Port=4
  __UniqueOutportName__1__ : Outport
  __UniqueOutportName__2__ : Outport  Port=2
  __UniqueOutportName__3__ : Outport  Port=3
  __UniqueOutportName__4__ : Outport  Port=4
  wires:
  Valve Vo2/1 -> __UniqueOutportName__4__/1
  Valve Vt/1 -> __UniqueOutportName__3__/1
  Valve Vo1/1 -> __UniqueOutportName__2__/1
  Pump/1 -> __UniqueOutportName__1__/1

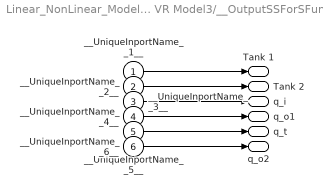
== system Linear_NonLinear_Model/COUPLED TANKS VR Model3/__OutputSSForSFun__ ==
  __UniqueInportName__1__ : Inport
  __UniqueInportName__2__ : Inport  Port=2
  __UniqueInportName__3__ : Inport  Port=3
  __UniqueInportName__4__ : Inport  Port=4
  __UniqueInportName__5__ : Inport  Port=5
  __UniqueInportName__6__ : Inport  Port=6
  Tank 1 : Outport  OutDataTypeStr=double  PortDimensions=1  SampleTime=[-1 0]
  Tank 2 : Outport  Port=2  OutDataTypeStr=double  PortDimensions=1  SampleTime=[-1 0]
  q_i : Outport  Port=3  OutDataTypeStr=double  PortDimensions=1  SampleTime=[0 1]
  q_o1 : Outport  Port=4  OutDataTypeStr=double  PortDimensions=1  SampleTime=[-1 0]
  q_t : Outport  Port=5  OutDataTypeStr=double  PortDimensions=1  SampleTime=[-1 0]
  q_o2 : Outport  Port=6  OutDataTypeStr=double  PortDimensions=1  SampleTime=[-1 0]
  wires:
  __UniqueInportName__6__/1 -> q_o2/1
  __UniqueInportName__5__/1 -> q_t/1
  __UniqueInportName__4__/1 -> q_o1/1
  __UniqueInportName__3__/1 -> q_i/1
  __UniqueInportName__2__/1 -> Tank 2/1
  __UniqueInportName__1__/1 -> Tank 1/1

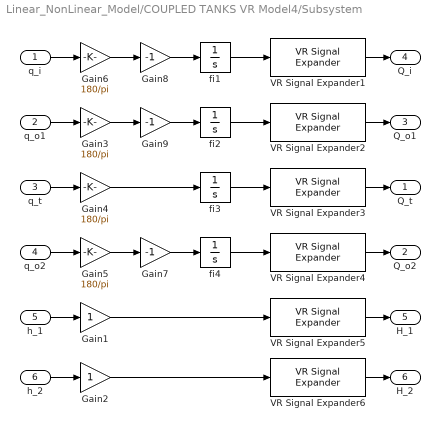
== system Linear_NonLinear_Model/COUPLED TANKS VR Model4/Subsystem ==
  q_i : Inport
  q_o1 : Inport  Port=2
  q_t : Inport  Port=3
  q_o2 : Inport  Port=4
  h_1 : Inport  Port=5
  h_2 : Inport  Port=6
  Gain1 : Gain
  Gain2 : Gain
  Gain{3..6} (4 alike) : Gain  Gain=180/pi
  Gain7 : Gain  Gain=-1
  Gain8 : Gain  Gain=-1
  Gain9 : Gain  Gain=-1
  VR Signal Expander{1..4} (4 alike) : vrlib/VR Signal Expander  outwidth=4  outidx=[4]
  VR Signal Expander5 : vrlib/VR Signal Expander  outwidth=3  outidx=[2]
  VR Signal Expander6 : vrlib/VR Signal Expander  outwidth=3  outidx=[2]
  fi{1..4} (4 alike) : Integrator
  Q_t : Outport
  Q_o2 : Outport  Port=2
  Q_o1 : Outport  Port=3
  Q_i : Outport  Port=4
  H_1 : Outport  Port=5
  H_2 : Outport  Port=6
  wires:
  Gain9/1 -> fi2/1
  Gain8/1 -> fi1/1
  Gain7/1 -> fi4/1
  Gain5/1 -> Gain7/1
  q_o2/1 -> Gain5/1
  VR Signal Expander4/1 -> Q_o2/1
  fi4/1 -> VR Signal Expander4/1
  Gain4/1 -> fi3/1
  Gain6/1 -> Gain8/1
  Gain3/1 -> Gain9/1
  q_t/1 -> Gain4/1
  q_o1/1 -> Gain3/1
  Gain2/1 -> VR Signal Expander6/1
  Gain1/1 -> VR Signal Expander5/1
  VR Signal Expander6/1 -> H_2/1
  VR Signal Expander5/1 -> H_1/1
  VR Signal Expander1/1 -> Q_i/1
  VR Signal Expander2/1 -> Q_o1/1
  VR Signal Expander3/1 -> Q_t/1
  h_2/1 -> Gain2/1
  h_1/1 -> Gain1/1
  q_i/1 -> Gain6/1
  fi2/1 -> VR Signal Expander2/1
  fi3/1 -> VR Signal Expander3/1
  fi1/1 -> VR Signal Expander1/1

== system Linear_NonLinear_Model/COUPLED TANKS VR Model4/__InputSSForSFun__ ==
  Pump : Inport
  Valve Vo1 : Inport  Port=2
  Valve Vt : Inport  Port=3
  Valve Vo2 : Inport  Port=4
  __UniqueOutportName__1__ : Outport
  __UniqueOutportName__2__ : Outport  Port=2
  __UniqueOutportName__3__ : Outport  Port=3
  __UniqueOutportName__4__ : Outport  Port=4
  wires:
  Valve Vo2/1 -> __UniqueOutportName__4__/1
  Valve Vt/1 -> __UniqueOutportName__3__/1
  Valve Vo1/1 -> __UniqueOutportName__2__/1
  Pump/1 -> __UniqueOutportName__1__/1

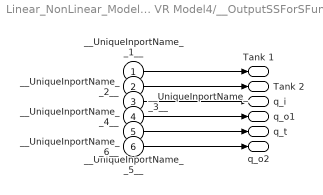
== system Linear_NonLinear_Model/COUPLED TANKS VR Model4/__OutputSSForSFun__ ==
  __UniqueInportName__1__ : Inport
  __UniqueInportName__2__ : Inport  Port=2
  __UniqueInportName__3__ : Inport  Port=3
  __UniqueInportName__4__ : Inport  Port=4
  __UniqueInportName__5__ : Inport  Port=5
  __UniqueInportName__6__ : Inport  Port=6
  Tank 1 : Outport  OutDataTypeStr=double  PortDimensions=1  SampleTime=[-1 0]
  Tank 2 : Outport  Port=2  OutDataTypeStr=double  PortDimensions=1  SampleTime=[-1 0]
  q_i : Outport  Port=3  OutDataTypeStr=double  PortDimensions=1  SampleTime=[0 1]
  q_o1 : Outport  Port=4  OutDataTypeStr=double  PortDimensions=1  SampleTime=[-1 0]
  q_t : Outport  Port=5  OutDataTypeStr=double  PortDimensions=1  SampleTime=[-1 0]
  q_o2 : Outport  Port=6  OutDataTypeStr=double  PortDimensions=1  SampleTime=[-1 0]
  wires:
  __UniqueInportName__6__/1 -> q_o2/1
  __UniqueInportName__5__/1 -> q_t/1
  __UniqueInportName__4__/1 -> q_o1/1
  __UniqueInportName__3__/1 -> q_i/1
  __UniqueInportName__2__/1 -> Tank 2/1
  __UniqueInportName__1__/1 -> Tank 1/1
